simulink model "majorprojectmodel"  (R2021a)
settings: Solver=VariableStepAuto  StartTime=0.0  StopTime=5  RelTol=1e-3
undefined symbols (not defined in the file): Ts
libraries: simulink x6, spsSeriesRLCBranchLib x5, spsIGBTLib x3, spsVoltageMeasurementLib x2, spspowerguiLib x2, spsDiodeLib x2, spsCurrentMeasurementLib x1, spsFuelCellStackLib x1, spsPermanentMagnetSynchronousMachineLib x1, spsThreePhaseVIMeasurementLib x1, spsUniversalBridgeLib x1
settings Model: Creator=Dell  LastModifiedBy=Dell

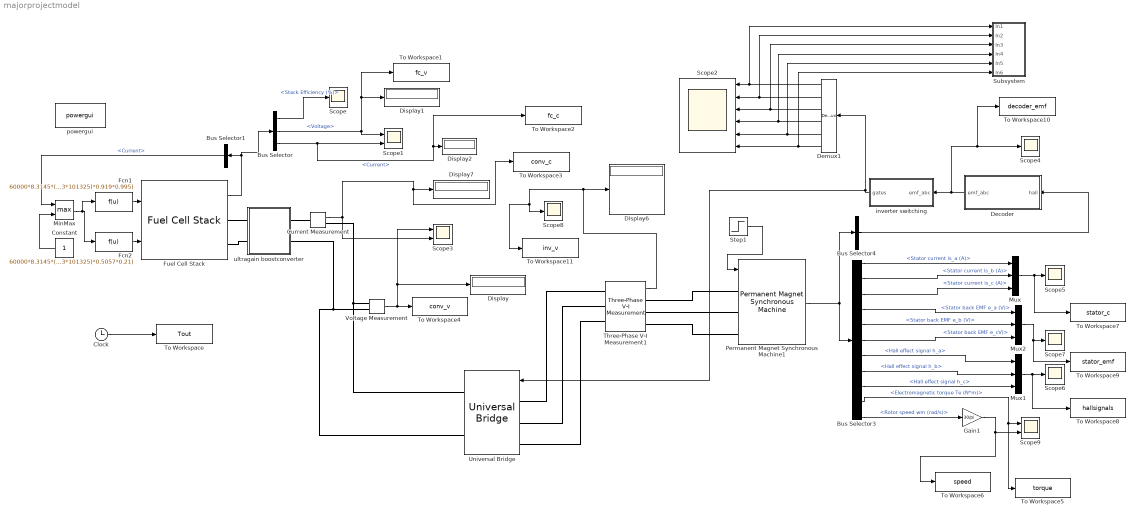
== system majorprojectmodel ==
  Bus Selector : BusSelector  OutputSignals=Stack Efficiency (%),Voltage,Current
  Bus Selector1 : BusSelector  OutputSignals=Current
  Bus Selector3 : BusSelector  OutputSignals=Stator current is_a (A),Stator current is_b (A),Stator current is_c (A),Stator back EMF e_a (V),Stator back EMF e_b (V),Stator back EMF e_cV),Hall effect signal h_a,Hall effect signal h_b,Hall effect signal h_c,Electromagnetic torque Te (N*m),Rotor speed wm (rad/s)
  Bus Selector4 : BusSelector  OutputSignals=Hall effect signal h_a,Hall effect signal h_b,Hall effect signal h_c  OutputAsBus=on
  Clock : Clock
  Constant : Constant
  Current Measurement : spsCurrentMeasurementLib/Current Measurement  PhasorSimulation=off  OutputType=Complex  PSBequivalent=0
  Decoder : Subsystem
  Demux1 : Demux  Outputs=6
  Display{,1..2,6..7} (5 alike) : Display
  Fcn1 : Fcn  Expr=60000*8.3145*(273+95)*400*u(1)/(2*96485*(3*101325)*0.919*0.995)
  Fcn2 : Fcn  Expr=60000*8.3145*(273+95)*400*u(1)/(4*96485*(3*101325)*0.5057*0.21)
  Fuel Cell Stack : spsFuelCellStackLib/Fuel Cell Stack  PresetModel=PEMFC - 1.26 kW - 24 Vdc  FcType=0  Detailed=Detailed  Eoc=[42,35]  NomVI=[52,24.23]  EndVI=[100,20]  Nc=42  n=46  TOp=55  AirFr=2400  SuppPress=[1.5,1]  Comp=[99.95,21,1]  SignX=off  SignY=off  FlowRateH2=on  FlowRateAir=on  SystemTemp=off  SystemPH2=off  SystemPAir=off  FCDyn=off  FC_tau=1  Peak_O2=80  V_Under=10
      settings: SourceProductBaseCode=PS
  Gain1 : Gain  Gain=30/pi
  MinMax : MinMax  Function=max  Inputs=2
  Mux : Mux  Inputs=3
  Mux1 : Mux  Inputs=3
  Mux2 : Mux  Inputs=3
  Permanent Magnet Synchronous Machine1 : spsPermanentMagnetSynchronousMachineLib/Permanent Magnet Synchronous Machine  NbPhases=3  FluxDistribution=Trapezoidal  RotorType=Round  MechanicalLoad=Torque Tm  PresetModel=No  ShowDetailedParameters=on  MeasurementBus=off  Resistance=1.43  Inductance=9.4e-3  dqInductances=[8.5e-3,8.5e-3]  La=0.000395  MachineConstant=Flux linkage established by magnets (V.s)  Flux=0.2158  VoltageCst=180.7882  TorqueCst=1.7264  Flat=120  Mechanical=[0.0027 0.0004924 4 0]  PolePairs=4  InitialConditions=[0,0, 0,0]  InitialConditions5ph=[0 0 0 0 0 0]  RefAngle=90 degrees behind phase A axis (modified Park)  IterativeDiscreteModel=Trapezoidal non iterative  TsBlock=-1  TsPowergui=0
  Scope{,4..8} (6 alike) : Scope
  Scope1 : Scope  NumInputPorts=2
  Scope2 : Scope  NumInputPorts=6
  Scope3 : Scope  NumInputPorts=2
  Scope9 : Scope  NumInputPorts=2
  Step1 : Step  Time=2.5  Before=5  After=10  SampleTime=0
  Subsystem : Subsystem
  Three-Phase V-I Measurement1 : spsThreePhaseVIMeasurementLib/Three-Phase V-I Measurement  VoltageMeasurement=phase-to-phase  SetLabelV=off  LabelV=Vabc  Vpu=off  VpuLL=off  CurrentMeasurement=no  SetLabelI=off  LabelI=Iabc  Ipu=off  Pbase=100e6  Vbase=500e3  OutputType=Complex  PhasorSimulation=off  PSBequivalent=0
  To Workspace : ToWorkspace  VariableName=Tout  SampleTime=Ts
      settings: Save2DSignal=2-D array (concatenate along first dimension)
  To Workspace1 : ToWorkspace  VariableName=fc_v  SampleTime=Ts
      settings: Save2DSignal=2-D array (concatenate along first dimension)
  To Workspace10 : ToWorkspace  VariableName=decoder_emf  SampleTime=Ts
      settings: Save2DSignal=2-D array (concatenate along first dimension)
  To Workspace11 : ToWorkspace  VariableName=inv_v  SampleTime=Ts
      settings: Save2DSignal=2-D array (concatenate along first dimension)
  To Workspace2 : ToWorkspace  VariableName=fc_c  SampleTime=Ts
      settings: Save2DSignal=2-D array (concatenate along first dimension)
  To Workspace3 : ToWorkspace  VariableName=conv_c  SampleTime=Ts
      settings: Save2DSignal=2-D array (concatenate along first dimension)
  To Workspace4 : ToWorkspace  VariableName=conv_v  SampleTime=Ts
      settings: Save2DSignal=2-D array (concatenate along first dimension)
  To Workspace5 : ToWorkspace  VariableName=torque  SampleTime=Ts
      settings: Save2DSignal=2-D array (concatenate along first dimension)
  To Workspace6 : ToWorkspace  VariableName=speed  SampleTime=Ts
      settings: Save2DSignal=2-D array (concatenate along first dimension)
  To Workspace7 : ToWorkspace  VariableName=stator_c  SampleTime=Ts
      settings: Save2DSignal=2-D array (concatenate along first dimension)
  To Workspace8 : ToWorkspace  VariableName=hallsignals  SampleTime=Ts
      settings: Save2DSignal=2-D array (concatenate along first dimension)
  To Workspace9 : ToWorkspace  VariableName=stator_emf  SampleTime=Ts
      settings: Save2DSignal=2-D array (concatenate along first dimension)
  Universal Bridge : spsUniversalBridgeLib/Universal Bridge  Arms=3  SnubberResistance=1e5  SnubberCapacitance=inf  Device=MOSFET / Diodes  Ron=1e-3  Lon=0  ForwardVoltages="[  0  0  ]"  ForwardVoltage=0  GTOparameters=[ 10e-6 , 20e-6 ]  IGBTparameters=[ 1e-6 , 2e-6 ]  Measurements=None  Measurements_2=None  converterType=Rectifier
  Voltage Measurement : spsVoltageMeasurementLib/Voltage Measurement  PhasorSimulation=off  OutputType=Complex  PSBequivalent=0
  inverter switching : Subsystem
  powergui : spspowerguiLib/powergui  Priority=1  SimulationMode=Discrete  SampleTime=Ts  frequency=60  Iterations=50  frequencyindice=0  Pbase=100e6  ErrMax=1e-4  UnitsV=kV  UnitsW=MW  buscounter=0  FunctionMessages=off  echomessages=off  EnableUseOfTLC=off  CurrentSourceSwitches=off  DisableSnubberDevices=off  DisableRonSwitches=off  DisableVfSwitches=off  DisplayEquations=off  AutomaticDiscreteSolvers=off  SolverType=Tustin/Backward Euler (TBE)  Interpol=off  ExternalGateDelay=off  methode=off  Ts=100  x0status=blocks  SPID=on  SwTol=0  HookPort=off  NonlinearTolerance=1e-4  nMaxIteration=100  ContinueOnMaxIteration=off  RestoreLinks=warning  ResistiveCurrentMeasurement=off  Frange=[0:2:500]  Ylog=off  Xlog=on  ShowGrid=off  save=off  variable=ZData  structure=0  ZoomFFT=off  StartTime=0.0  cycles=1  DisplayStyle=1  fundamental=60  FreqAxis=off  MaxFrequency=1000  frequencyindicesteady=1  RmsSteady=1  display=off
  ultragain boostconverter : Subsystem
  wires:
  Current Measurement/1 -> To Workspace3/1, Display7/1, Scope3/2
  Bus Selector3/6 -> Mux2/3  "<Stator back EMF e_cV)>"
  Three-Phase V-I Measurement1/1 -> To Workspace11/1, Scope8/1, Display6/1
  Bus Selector3/2 -> Mux/2  "<Stator current is_b (A)>"
  Bus Selector3/10 -> To Workspace5/1, Scope9/1  "<Electromagnetic torque Te (N*m)>"
  Bus Selector4/1 -> Decoder/1(hall)
  Bus Selector3/9 -> Mux1/3  "<Hall effect signal h_c>"
  Bus Selector/1 -> Scope/1  "<Stack Efficiency (%)>"
  Decoder/1(emf_abc) -> To Workspace10/1, Scope4/1, inverter switching/1(emf_abc)
  Bus Selector3/3 -> Mux/3  "<Stator current is_c (A)>"
  Bus Selector3/4 -> Mux2/1  "<Stator back EMF e_a (V)>"
  Voltage Measurement/1 -> Scope3/1, Display/1, To Workspace4/1
  Fcn2/1 -> Fuel Cell Stack/2
  Bus Selector/3 -> Scope1/2, To Workspace2/1, Display2/1  "<Current>"
  Fcn1/1 -> Fuel Cell Stack/1
  Gain1/1 -> To Workspace6/1, Scope9/2
  Bus Selector3/11 -> Gain1/1  "<Rotor speed wm (rad/s)>"
  inverter switching/1(gates) -> Universal Bridge/1, Demux1/1
  Permanent Magnet Synchronous Machine1/1 -> Bus Selector4/1, Bus Selector3/1
  Bus Selector3/7 -> Mux1/1  "<Hall effect signal h_a>"
  Bus Selector3/8 -> Mux1/2  "<Hall effect signal h_b>"
  Bus Selector3/1 -> Mux/1  "<Stator current is_a (A)>"
  Fuel Cell Stack/1 -> Bus Selector/1, Bus Selector1/1
  Constant/1 -> MinMax/2
  MinMax/1 -> Fcn1/1, Fcn2/1
  Bus Selector/2 -> To Workspace1/1, Display1/1, Scope1/1  "<Voltage>"
  Bus Selector3/5 -> Mux2/2  "<Stator back EMF e_b (V)>"
  Bus Selector1/1 -> MinMax/1  "<Current>"
  Demux1/5 -> Subsystem/5(In5), Scope2/5
  Demux1/6 -> Subsystem/6(In6), Scope2/6
  Clock/1 -> To Workspace/1
  Mux/1 -> To Workspace7/1, Scope5/1
  Mux1/1 -> To Workspace8/1, Scope6/1
  Step1/1 -> Permanent Magnet Synchronous Machine1/1
  Mux2/1 -> To Workspace9/1, Scope7/1
  Demux1/1 -> Subsystem/1(In1), Scope2/1
  Demux1/2 -> Subsystem/2(In2), Scope2/2
  Demux1/3 -> Subsystem/3(In3), Scope2/3
  Demux1/4 -> Subsystem/4(In4), Scope2/4
  connections:
  Current Measurement/RConn1 -- Universal Bridge/RConn1 -- Voltage Measurement/LConn1
  Three-Phase V-I Measurement1/RConn1 -- Permanent Magnet Synchronous Machine1/LConn1
  Universal Bridge/LConn2 -- Three-Phase V-I Measurement1/LConn2
  Universal Bridge/LConn3 -- Three-Phase V-I Measurement1/LConn3
  Three-Phase V-I Measurement1/RConn3 -- Permanent Magnet Synchronous Machine1/LConn3
  Three-Phase V-I Measurement1/RConn2 -- Permanent Magnet Synchronous Machine1/LConn2
  Universal Bridge/LConn1 -- Three-Phase V-I Measurement1/LConn1
  Universal Bridge/RConn2 -- ultragain boostconverter/RConn2 -- Voltage Measurement/LConn2
  ultragain boostconverter/LConn1 -- Fuel Cell Stack/RConn1
  Fuel Cell Stack/RConn2 -- ultragain boostconverter/LConn2
  ultragain boostconverter/RConn1 -- Current Measurement/LConn1

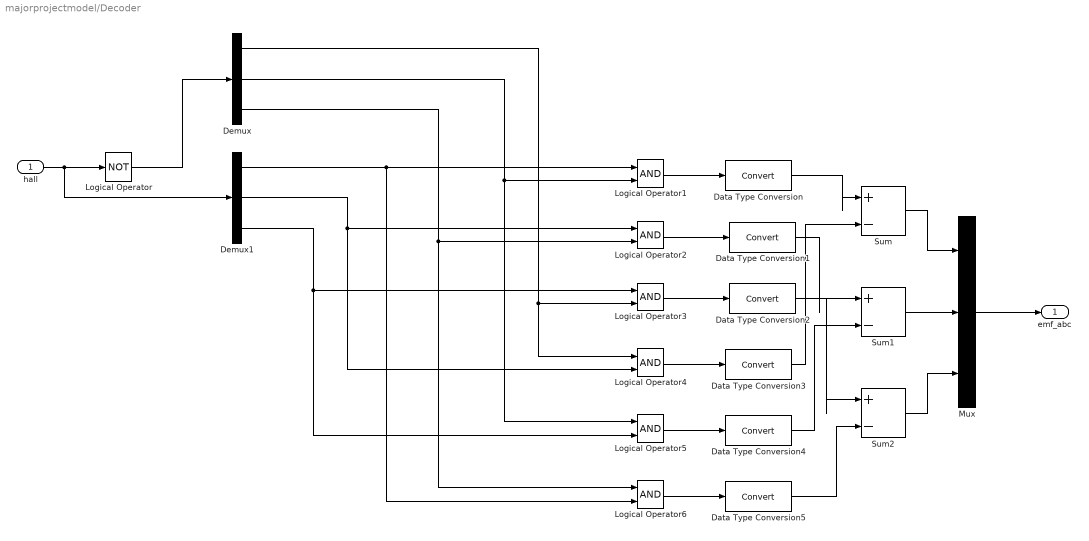
== system majorprojectmodel/Decoder ==
  hall : Inport
  Data Type Conversion{,1..5} (6 alike) : DataTypeConversion
  Demux : Demux  Outputs=3
  Demux1 : Demux  Outputs=3
  Logical Operator : Logic  Operator=NOT  AllPortsSameDT=off  OutDataTypeStr=boolean
  Logical Operator{1..6} (6 alike) : Logic  AllPortsSameDT=off  OutDataTypeStr=boolean
  Mux : Mux  Inputs=3
  Sum : Sum  Inputs=|+-
  Sum1 : Sum  Inputs=|+-
  Sum2 : Sum  Inputs=|+-
  emf_abc : Outport
  wires:
  hall/1 -> Demux1/1, Logical Operator/1
  Logical Operator1/1 -> Data Type Conversion/1
  Logical Operator2/1 -> Data Type Conversion1/1
  Logical Operator3/1 -> Data Type Conversion2/1
  Logical Operator4/1 -> Data Type Conversion3/1
  Logical Operator5/1 -> Data Type Conversion4/1
  Logical Operator6/1 -> Data Type Conversion5/1
  Data Type Conversion/1 -> Sum/1
  Data Type Conversion1/1 -> Sum1/1
  Data Type Conversion2/1 -> Sum2/1
  Data Type Conversion3/1 -> Sum/2
  Data Type Conversion4/1 -> Sum1/2
  Data Type Conversion5/1 -> Sum2/2
  Sum/1 -> Mux/1
  Sum1/1 -> Mux/2
  Sum2/1 -> Mux/3
  Mux/1 -> emf_abc/1
  Logical Operator/1 -> Demux/1
  Demux1/1 -> Logical Operator6/2, Logical Operator1/1
  Demux/1 -> Logical Operator3/2, Logical Operator4/1
  Demux/2 -> Logical Operator1/2, Logical Operator5/1
  Demux/3 -> Logical Operator6/1, Logical Operator2/2
  Demux1/2 -> Logical Operator2/1, Logical Operator4/2
  Demux1/3 -> Logical Operator3/1, Logical Operator5/2

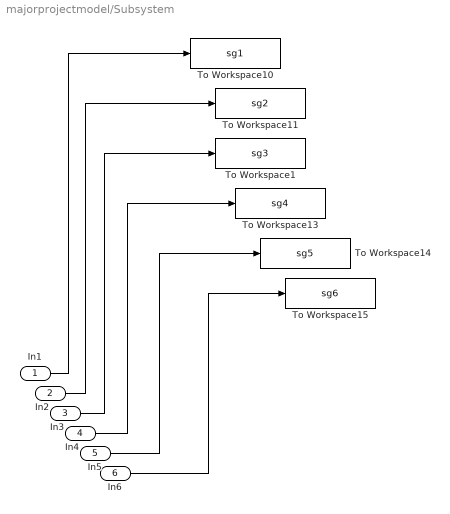
== system majorprojectmodel/Subsystem ==
  In1 : Inport
  In2 : Inport  Port=2
  In3 : Inport  Port=3
  In4 : Inport  Port=4
  In5 : Inport  Port=5
  In6 : Inport  Port=6
  To Workspace1 : ToWorkspace  VariableName=sg3  SampleTime=Ts
      settings: Save2DSignal=2-D array (concatenate along first dimension)
  To Workspace10 : ToWorkspace  VariableName=sg1  SampleTime=Ts
      settings: Save2DSignal=2-D array (concatenate along first dimension)
  To Workspace11 : ToWorkspace  VariableName=sg2  SampleTime=Ts
      settings: Save2DSignal=2-D array (concatenate along first dimension)
  To Workspace13 : ToWorkspace  VariableName=sg4  SampleTime=Ts
      settings: Save2DSignal=2-D array (concatenate along first dimension)
  To Workspace14 : ToWorkspace  VariableName=sg5  SampleTime=Ts
      settings: Save2DSignal=2-D array (concatenate along first dimension)
  To Workspace15 : ToWorkspace  VariableName=sg6  SampleTime=Ts
      settings: Save2DSignal=2-D array (concatenate along first dimension)
  wires:
  In5/1 -> To Workspace14/1
  In3/1 -> To Workspace1/1
  In1/1 -> To Workspace10/1
  In6/1 -> To Workspace15/1
  In4/1 -> To Workspace13/1
  In2/1 -> To Workspace11/1

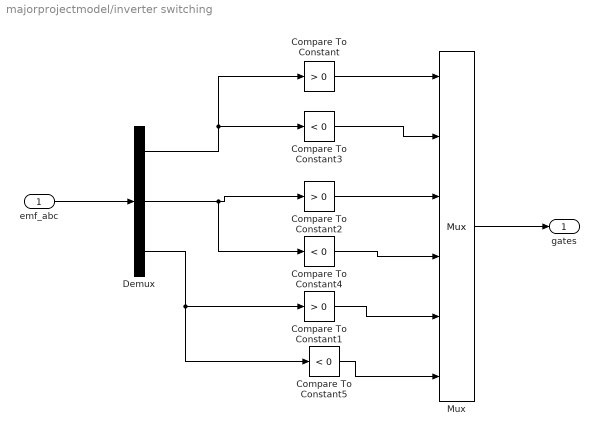
== system majorprojectmodel/inverter switching ==
  emf_abc : Inport
  Compare To Constant : simulink/Logic and Bit Operations/Compare To Constant  relop=>  const=0  OutDataTypeStr=boolean
  Compare To Constant1 : simulink/Logic and Bit Operations/Compare To Constant  relop=>  const=0  OutDataTypeStr=boolean
  Compare To Constant2 : simulink/Logic and Bit Operations/Compare To Constant  relop=>  const=0  OutDataTypeStr=boolean
  Compare To Constant3 : simulink/Logic and Bit Operations/Compare To Constant  relop=<  const=0  OutDataTypeStr=boolean
  Compare To Constant4 : simulink/Logic and Bit Operations/Compare To Constant  relop=<  const=0  OutDataTypeStr=boolean
  Compare To Constant5 : simulink/Logic and Bit Operations/Compare To Constant  relop=<  const=0  OutDataTypeStr=boolean
  Demux : Demux  Outputs=3
  Mux : Mux  Inputs=6
  gates : Outport
  wires:
  emf_abc/1 -> Demux/1
  Demux/1 -> Compare To Constant3/1, Compare To Constant/1
  Demux/2 -> Compare To Constant4/1, Compare To Constant2/1
  Demux/3 -> Compare To Constant5/1, Compare To Constant1/1
  Compare To Constant/1 -> Mux/1
  Compare To Constant3/1 -> Mux/2
  Compare To Constant2/1 -> Mux/3
  Compare To Constant4/1 -> Mux/4
  Compare To Constant1/1 -> Mux/5
  Compare To Constant5/1 -> Mux/6
  Mux/1 -> gates/1

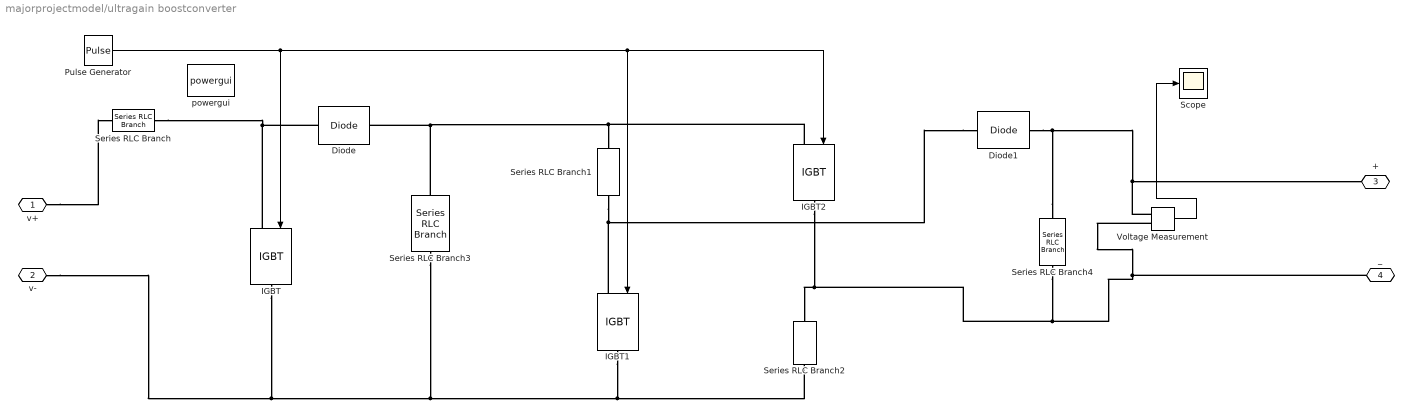
== system majorprojectmodel/ultragain boostconverter ==
  Diode : spsDiodeLib/Diode  Ron=0.01  Lon=0  Vf=0.3  IC=0  UseSnubber=off  Rs=50000  Cs=250e-9  Measurements=off
  Diode1 : spsDiodeLib/Diode  Ron=0.01  Lon=0  Vf=0.3  IC=0  UseSnubber=off  Rs=50000  Cs=250e-9  Measurements=off
  IGBT : spsIGBTLib/IGBT  Ron=0.001  Lon=0  Vf=1  Tf=1e-6  Tt=2e-6  IC=0  Rs=1e5  Cs=inf  Measurements=off
  IGBT1 : spsIGBTLib/IGBT  Ron=0.001  Lon=0  Vf=1  Tf=1e-6  Tt=2e-6  IC=0  Rs=1e5  Cs=inf  Measurements=off
  IGBT2 : spsIGBTLib/IGBT  Ron=0.001  Lon=0  Vf=1  Tf=1e-6  Tt=2e-6  IC=0  Rs=1e5  Cs=inf  Measurements=off
  Pulse Generator : DiscretePulseGenerator  PulseType=Time based  Period=1/30000  PulseWidth=34
  Scope : Scope
  Series RLC Branch : spsSeriesRLCBranchLib/Series RLC Branch  LConnTagsString=__new0  RConnTagsString=__new0  BranchType=L  Resistance=1  Inductance=3e-3  SetiL0=off  InitialCurrent=0  Capacitance=1e-6  Setx0=off  InitialVoltage=0  Measurements=None
  Series RLC Branch1 : spsSeriesRLCBranchLib/Series RLC Branch  LConnTagsString=__new0  RConnTagsString=__new0  BranchType=L  Resistance=1  Inductance=3e-3  SetiL0=off  InitialCurrent=0  Capacitance=1e-6  Setx0=off  InitialVoltage=0  Measurements=None
  Series RLC Branch2 : spsSeriesRLCBranchLib/Series RLC Branch  LConnTagsString=__new0  RConnTagsString=__new0  BranchType=L  Resistance=1  Inductance=3e-3  SetiL0=off  InitialCurrent=0  Capacitance=1e-6  Setx0=off  InitialVoltage=0  Measurements=None
  Series RLC Branch3 : spsSeriesRLCBranchLib/Series RLC Branch  LConnTagsString=__new0  RConnTagsString=__new0  BranchType=C  Resistance=1  Inductance=1e-3  SetiL0=off  InitialCurrent=0  Capacitance=260e-6  Setx0=off  InitialVoltage=0  Measurements=None
  Series RLC Branch4 : spsSeriesRLCBranchLib/Series RLC Branch  LConnTagsString=__new0  RConnTagsString=__new0  BranchType=C  Resistance=1  Inductance=1e-3  SetiL0=off  InitialCurrent=0  Capacitance=260e-6  Setx0=off  InitialVoltage=0  Measurements=None
  Voltage Measurement : spsVoltageMeasurementLib/Voltage Measurement  PhasorSimulation=off  OutputType=Complex  PSBequivalent=0
  powergui : spspowerguiLib/powergui  Priority=1  SimulationMode=Continuous  SampleTime=1e-5  frequency=60  Iterations=50  frequencyindice=0  Pbase=100e6  ErrMax=1e-4  UnitsV=kV  UnitsW=MW  buscounter=0  FunctionMessages=off  echomessages=off  EnableUseOfTLC=off  CurrentSourceSwitches=off  DisableSnubberDevices=off  DisableRonSwitches=off  DisableVfSwitches=off  DisplayEquations=off  AutomaticDiscreteSolvers=off  SolverType=Tustin/Backward Euler (TBE)  Interpol=off  ExternalGateDelay=off  methode=off  Ts=100  x0status=blocks  SPID=on  SwTol=0  HookPort=off  NonlinearTolerance=1e-4  nMaxIteration=100  ContinueOnMaxIteration=off  RestoreLinks=warning  ResistiveCurrentMeasurement=off  Frange=[0:2:500]  Ylog=off  Xlog=on  ShowGrid=off  save=off  variable=ZData  structure=0  ZoomFFT=off  StartTime=0.0  cycles=1  DisplayStyle=1  fundamental=60  FreqAxis=off  MaxFrequency=1000  frequencyindicesteady=1  RmsSteady=1  display=off
  v+ : PMIOPort  Side=Left
  v- : PMIOPort  Port=2  Side=Left
  + : PMIOPort  Port=3  Side=Right
  _ : PMIOPort  Port=4  Side=Right
  wires:
  Pulse Generator/1 -> IGBT/1, IGBT2/1, IGBT1/1
  Voltage Measurement/1 -> Scope/1
  connections:
  v+/RConn1 -- Series RLC Branch/LConn1
  Series RLC Branch/RConn1 -- IGBT/LConn1 -- Diode/LConn1
  Diode1/LConn1 -- IGBT1/LConn1 -- Series RLC Branch1/RConn1
  Series RLC Branch4/LConn1 -- Diode1/RConn1 -- +/RConn1 -- Voltage Measurement/LConn1
  Voltage Measurement/LConn2 -- _/RConn1 -- Series RLC Branch4/RConn1 -- IGBT2/RConn1 -- Series RLC Branch2/LConn1
  Series RLC Branch3/LConn1 -- Diode/RConn1 -- IGBT2/LConn1 -- Series RLC Branch1/LConn1
  Series RLC Branch2/RConn1 -- IGBT1/RConn1 -- IGBT/RConn1 -- v-/RConn1 -- Series RLC Branch3/RConn1
